simulink model "Junctions1"  (R2020a)
settings: Solver=VariableStepAuto  StartTime=0.0  StopTime=0.1  RelTol=1e-3
settings Model: Creator=86188  LastModifiedBy=bzhan
settings DataIOCC: ReturnWorkspaceOutputs=off
settings DebuggingCC: ArithmeticOperatorsInVariantConditions=warning
settings SFSimCC: SimUseLocalCustomCode=off  CustomCodeUndefinedFunction=UseInterfaceOnly
settings RTWCC: RTWUseLocalCustomCode=off

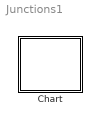
== system Junctions1 ==
  Chart : Stateflow chart  TreatAsAtomicUnit=on

== stateflow chart Junctions1/Chart ==
  settings: updateMethod=DISCRETE  sampleTime=0.1
  state B
    en: f("enB")
  state A
    en: f("enA")
    du: f("duA")
  state C
    en: f("enC")
  state E
    en: f("enE")
  state D
    en: f("enD")
  (junction 3) -> B [order 1] : [y>10]
  (default) -> A : {y=4;}
  A -> (junction 3)
  (junction 3) -> C [order 2] : [y>5]
  (junction 3) -> E [order 4] : [y>=1]
  (junction 3) -> D [order 3] : [y>3]
  data: s function_input; y local
  function f(s):
    | function f(s)
    |   fprintf(s+"\n");
